simulink model "Energy_Management"  (R2025a)
settings: Solver=ode23tb  StartTime=0.0  StopTime=0.5  MaxStep=1e-5  RelTol=1e-3
undefined symbols (not defined in the file): Ion, Lithium
libraries: eeDiscretePi x7, spsSeriesRLCBranchLib x7, spsCurrentMeasurementLib x4, spsIGBTDiodeLib x4, spsPWMGeneratorDCDCLib x3, spsVoltageMeasurementLib x3, spsDiodeLib x2, spsBatteryLib x1, spsFuelCellStackLib x1, spsPVArrayLib x1, spsPWMGenerator2LevelLib x1, spsSeriesRLCLoadLib x1
settings Model: Creator=devin  LastModifiedBy=devin

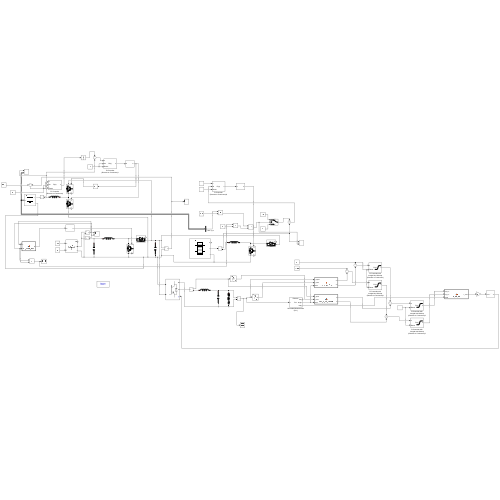
[thumbnail: Simulink's stored preview of the top-level diagram]
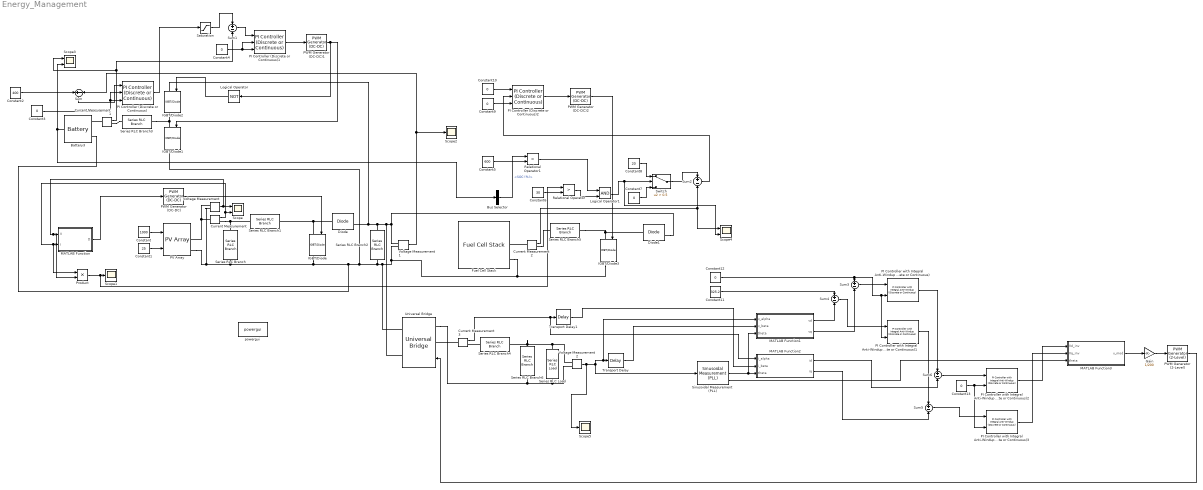
== system Energy_Management ==
  Battery3 : spsBatteryLib/Battery  BatType=Lithium-Ion  NomV=300  NomQ=48  SOC=100  Batt_Tr=45  PresetModel=on  MaxQ=48  MinV=225  FullV=349.1961  Dis_rate=20.8696  R=0.0625  Normal_OP=43.4087  expZone="[324.1158      2.358261]"
  Bus Selector : BusSelector  OutputSignals=SOC (%)
  Constant : Constant  Value=1000
  Constant1 : Constant  Value=25
  Constant{3..4,7,9..10,12..13} (7 alike) : Constant  Value=0
  Constant11 : Constant  Value=325.2
  Constant2 : Constant  Value=400
  Constant5 : Constant  Value=600
  Constant6 : Constant  Value=30
  Constant8 : Constant  Value=20
  Current Measurement{,1..3} (4 alike) : spsCurrentMeasurementLib/Current Measurement  PhasorSimulation=off  OutputType=Complex  PSBequivalent=0
  Diode : spsDiodeLib/Diode  Ron=0.001  Lon=0  Vf=0.8  IC=0  UseSnubber=0  Rs=500  Cs=250e-9  Measurements=on
  Diode1 : spsDiodeLib/Diode  Ron=0.001  Lon=0  Vf=0.8  IC=0  UseSnubber=0  Rs=500  Cs=250e-9  Measurements=on
  Fuel Cell Stack : spsFuelCellStackLib/Fuel Cell Stack  PresetModel=No (User-Defined)  FcType=0  Detailed=Detailed  Eoc=[330, 300]  NomVI=[20, 220]  EndVI=[35, 200]  Nc=315  n=55  TOp=65  AirFr=300  SuppPress=[1.5,1]  Comp=[99.95,21,1]  SignX=off  SignY=off  FlowRateH2=off  FlowRateAir=off  SystemTemp=off  SystemPH2=off  SystemPAir=off  FCDyn=off  FC_tau=1  Peak_O2=80  V_Under=10
      settings: LibrarySourceBlock=sps_lib/Sources/Fuel Cell Stack
  Gain : Gain  Gain=1/200
  IGBT/Diode{,1..3} (4 alike) : spsIGBTDiodeLib/IGBT//Diode  Ron=1e-3  Rs=1e5  Cs=inf  Measurements=on
  Logical Operator : Logic  Operator=NOT  AllPortsSameDT=off  OutDataTypeStr=boolean
  Logical Operator1 : Logic  AllPortsSameDT=off  OutDataTypeStr=boolean
  MATLAB Function : MATLAB Function  TreatAsAtomicUnit=on
  MATLAB Function1 : MATLAB Function  TreatAsAtomicUnit=on
  MATLAB Function2 : MATLAB Function  TreatAsAtomicUnit=on
  MATLAB Function3 : MATLAB Function  TreatAsAtomicUnit=on
  PI Controller (Discrete or Continuous) : eeDiscretePi/PI Controller (Discrete or Continuous)  Kp=0.1  Ki=5  Kaw=1  x0=0  Ts=-1
      settings: LibrarySourceBlock=|
      | ee_sl_lib/General Control/PI Controller
      | (Discrete or Continuous)
  PI Controller (Discrete or Continuous)1 : eeDiscretePi/PI Controller (Discrete or Continuous)  Kp=0.1  Ki=5  Kaw=1  x0=0  Ts=-1
      settings: LibrarySourceBlock=|
      | ee_sl_lib/General Control/PI Controller
      | (Discrete or Continuous)
  PI Controller (Discrete or Continuous)2 : eeDiscretePi/PI Controller (Discrete or Continuous)  Kp=0.2  Ki=20  Kaw=1  x0=0  Ts=-1
      settings: LibrarySourceBlock=|
      | ee_sl_lib/General Control/PI Controller
      | (Discrete or Continuous)
  PI Controller with Integral Anti-Windup (Discrete or Continuous) : eeDiscretePi/PI Controller with Integral Anti-Windup (Discrete or Continuous)  Kp=0.2  Ki=25  x0=0  B=15  A=-15  Ts=-1
      settings: LibrarySourceBlock=|
      | ee_sl_lib/General Control/PI Controller with
      | Integral Anti-Windup
      | (Discrete or Continuous)
  PI Controller with Integral Anti-Windup (Discrete or Continuous)1 : eeDiscretePi/PI Controller with Integral Anti-Windup (Discrete or Continuous)  Kp=0.2  Ki=25  x0=0  B=15  A=-15  Ts=-1
      settings: LibrarySourceBlock=|
      | ee_sl_lib/General Control/PI Controller with
      | Integral Anti-Windup
      | (Discrete or Continuous)
  PI Controller with Integral Anti-Windup (Discrete or Continuous)2 : eeDiscretePi/PI Controller with Integral Anti-Windup (Discrete or Continuous)  Kp=0.4  Ki=40  x0=0  B=0.95  A=-0.95  Ts=-1
      settings: LibrarySourceBlock=|
      | ee_sl_lib/General Control/PI Controller with
      | Integral Anti-Windup
      | (Discrete or Continuous)
  PI Controller with Integral Anti-Windup (Discrete or Continuous)3 : eeDiscretePi/PI Controller with Integral Anti-Windup (Discrete or Continuous)  Kp=0.4  Ki=40  x0=0  B=0.95  A=-0.95  Ts=-1
      settings: LibrarySourceBlock=|
      | ee_sl_lib/General Control/PI Controller with
      | Integral Anti-Windup
      | (Discrete or Continuous)
  PV Array : spsPVArrayLib/PV Array  Npar=1  Nser=8  PlotType=array @ 1000 W/m2 & specified temperatures  S_vec="[ 1000  500  100 ]"  Temp_C_vec="[ 45 25  ]"  ModuleName=User-defined  PlotWhenSelected=off  Pm=250.205  Ncell=60  Voc=37.8  Isc=8.75  Vm=30.7  Im=8.15  beta_Voc_pc=-0.36099  alpha_Isc_pc=0.102  beta_Voc=-0.13645  alpha_Isc=0.008925  IL=8.764  I0=3.2541e-10  nI=1.0219  Rsh=197.3099  Rs=0.29997  RobustModel=off  RobustCellTemperature=313.3991  BAL=on  Tc=1e-6  Tfilter=5e-5
  PWM Generator (2-Level) : spsPWMGenerator2LevelLib/PWM Generator (2-Level)  ModulatorType=Single-phase full-bridge - Bipolar modulation (4 pulses)  ModulatorMode=Unsynchronized  Fc=1000  Pc=90  nF=27  MinMax="[ -1  1 ]"  SamplingTechnique=Natural  ModulatingSignals=off  m=0.8  Freq=60  Phase=0  Ts=0  ShowCarrierOutport=off
  PWM Generator (DC-DC) : spsPWMGeneratorDCDCLib/PWM Generator (DC-DC)  Fsw=20000  Ts=0
  PWM Generator (DC-DC)1 : spsPWMGeneratorDCDCLib/PWM Generator (DC-DC)  Fsw=20000  Ts=0
  PWM Generator (DC-DC)2 : spsPWMGeneratorDCDCLib/PWM Generator (DC-DC)  Fsw=20000  Ts=0
  Product : Product
  Relational Operator : RelationalOperator  Operator=>  OutDataTypeStr=boolean  RndMeth=Simplest  InputSameDT=off
  Relational Operator1 : RelationalOperator  Operator=>  OutDataTypeStr=boolean  RndMeth=Simplest  InputSameDT=off
  Saturation : Saturate  UpperLimit=0.95  LowerLimit=0.05
  Scope : Scope  NumInputPorts=2
      settings: ActiveDisplayYMinimum=-32.437505931636437  ActiveDisplayYMaximum=299.72938020086377
  Scope1 : Scope
      settings: ActiveDisplayYMinimum=-250.09653918436439  ActiveDisplayYMaximum=2251.6858311968886
  Scope2 : Scope
      settings: ActiveDisplayYMinimum=327.296191460694  ActiveDisplayYMaximum=408.0782422570619  DataLoggingVariableName=ScopeData2
  Scope3 : Scope  NumInputPorts=2
      settings: ActiveDisplayYMinimum=-49.354169180280678  ActiveDisplayYMaximum=395.26293627147709  DataLoggingVariableName=ScopeData3
  Scope4 : Scope  NumInputPorts=2
      settings: ActiveDisplayYMinimum=-0.17740712010289458  ActiveDisplayYMaximum=0.30140270835281957  DataLoggingVariableName=ScopeData4
  Scope5 : Scope
      settings: ActiveDisplayYMinimum=-2463.1886461096151  ActiveDisplayYMaximum=2405.0943637829546  DataLoggingVariableName=ScopeData5
  Series RLC Branch : spsSeriesRLCBranchLib/Series RLC Branch  LConnTagsString=__new0  RConnTagsString=__new0  BranchType=C  Resistance=1  Inductance=1e-3  SetiL0=off  InitialCurrent=0  Capacitance=470e-6  Setx0=off  InitialVoltage=0  Measurements=None
  Series RLC Branch1 : spsSeriesRLCBranchLib/Series RLC Branch  LConnTagsString=__new0  RConnTagsString=__new0  BranchType=L  Resistance=1  Inductance=1e-3  SetiL0=off  InitialCurrent=0  Capacitance=1e-6  Setx0=off  InitialVoltage=0  Measurements=None
  Series RLC Branch2 : spsSeriesRLCBranchLib/Series RLC Branch  LConnTagsString=__new0  RConnTagsString=__new0  BranchType=C  Resistance=1  Inductance=1e-3  SetiL0=off  InitialCurrent=0  Capacitance=2200e-6  Setx0=on  InitialVoltage=400  Measurements=None
  Series RLC Branch3 : spsSeriesRLCBranchLib/Series RLC Branch  LConnTagsString=__new0  RConnTagsString=__new0  BranchType=L  Resistance=1  Inductance=2e-3  SetiL0=off  InitialCurrent=0  Capacitance=1e-6  Setx0=off  InitialVoltage=0  Measurements=None
  Series RLC Branch4 : spsSeriesRLCBranchLib/Series RLC Branch  LConnTagsString=__new0  RConnTagsString=__new0  BranchType=L  Resistance=1  Inductance=2e-3  SetiL0=off  InitialCurrent=0  Capacitance=1e-6  Setx0=off  InitialVoltage=0  Measurements=None
  Series RLC Branch5 : spsSeriesRLCBranchLib/Series RLC Branch  LConnTagsString=__new0  RConnTagsString=__new0  BranchType=L  Resistance=1  Inductance=1e-3  SetiL0=off  InitialCurrent=0  Capacitance=1e-6  Setx0=off  InitialVoltage=0  Measurements=None
  Series RLC Branch6 : spsSeriesRLCBranchLib/Series RLC Branch  LConnTagsString=__new0  RConnTagsString=__new0  BranchType=C  Resistance=1  Inductance=2e-3  SetiL0=off  InitialCurrent=0  Capacitance=10e-6  Setx0=off  InitialVoltage=0  Measurements=None
  Series RLC Load : spsSeriesRLCLoadLib/Series RLC Load  LConnTagsString=a  RConnTagsString=__new0  NominalVoltage=230  NominalFrequency=50  ActivePower=1200  InductivePower=100  CapacitivePower=100  Setx0=off  InitialVoltage=0  SetiL0=off  InitialCurrent=0  Measurements=None  LoadType=constant Z
  Sinusoidal Measurement (PLL) : eeSinusoidalMeasurementV2/Sinusoidal Measurement (PLL)  Ki_PD=1000  Kp_LF=400  Ki_LF=20000  F0=50  Theta0=0  Mag0=1  Ts=1e-6
      settings: LibrarySourceBlock=|
      | ee_sl_lib/Measurements/Sinusoidal Measurement
      | (PLL)
  Sum{,1..6} (7 alike) : Sum  Inputs=+-
  Switch : Switch  Criteria=u2 > Threshold  Threshold=0.5  SaturateOnIntegerOverflow=off  InputSameDT=off
  Transport Delay : TransportDelay  DelayTime=0.005  BufferSize=8192
  Transport Delay1 : TransportDelay  DelayTime=0.005  BufferSize=8192
  Universal Bridge : spsUniversalBridgeLib/Universal Bridge  Arms=2  SnubberResistance=1e5  SnubberCapacitance=inf  Device=IGBT / Diodes  Ron=1e-3  Lon=0  ForwardVoltages="[  0  0  ]"  ForwardVoltage=0  GTOparameters=[ 10e-6 , 20e-6 ]  IGBTparameters=[ 1e-6 , 2e-6 ]  Measurements=None  Measurements_2=None  converterType=Rectifier
  Voltage Measurement : spsVoltageMeasurementLib/Voltage Measurement  PhasorSimulation=off  OutputType=Complex  PSBequivalent=0
  Voltage Measurement1 : spsVoltageMeasurementLib/Voltage Measurement  PhasorSimulation=off  OutputType=Complex  PSBequivalent=0
  Voltage Measurement2 : spsVoltageMeasurementLib/Voltage Measurement  PhasorSimulation=off  OutputType=Complex  PSBequivalent=0
  powergui : sps_lib/powergui  Priority=1  SimulationMode=Discrete  SampleTime=1e-6  frequency=60  Iterations=50  frequencyindice=0  Pbase=100e6  ErrMax=1e-4  UnitsV=kV  UnitsW=MW  buscounter=0  FunctionMessages=off  echomessages=off  EnableUseOfTLC=off  CurrentSourceSwitches=off  DisableSnubberDevices=off  DisableRonSwitches=off  DisableVfSwitches=off  DisplayEquations=off  AutomaticDiscreteSolvers=off  SolverType=Tustin/Backward Euler (TBE)  Interpol=off  ExternalGateDelay=off  methode=off  Ts=100  x0status=blocks  SPID=on  SwTol=0  HookPort=off  NonlinearTolerance=1e-4  nMaxIteration=100  ContinueOnMaxIteration=off  RestoreLinks=warning  ResistiveCurrentMeasurement=off  Frange=[0:2:500]  Ylog=off  Xlog=on  ShowGrid=off  save=off  variable=ZData  structure=0  ZoomFFT=off  StartTime=0.0  cycles=1  DisplayStyle=1  fundamental=60  FreqAxis=off  MaxFrequency=1000  frequencyindicesteady=1  RmsSteady=1  display=off
  wires:
  Voltage Measurement/1 -> Product/2, MATLAB Function/1(V), Scope/1
  Current Measurement/1 -> Product/1, MATLAB Function/2(I), Scope/2
  MATLAB Function/1(D) -> PWM Generator (DC-DC)/1
  PWM Generator (DC-DC)/1 -> IGBT/Diode/1
  Constant/1 -> PV Array/1
  Constant1/1 -> PV Array/2
  Constant2/1 -> Sum/1
  Voltage Measurement1/1 -> Sum/2, Scope2/1
  Sum/1 -> PI Controller (Discrete or Continuous)/1
  PI Controller (Discrete or Continuous)/1 -> Saturation/1
  PWM Generator (DC-DC)1/1 -> Logical Operator/1, IGBT/Diode1/1
  Logical Operator/1 -> IGBT/Diode2/1
  Constant3/1 -> PI Controller (Discrete or Continuous)/3, PI Controller (Discrete or Continuous)/2
  Saturation/1 -> Sum1/1
  Current Measurement1/1 -> Sum1/2, Scope3/1
  PI Controller (Discrete or Continuous)1/1 -> PWM Generator (DC-DC)1/1
  Sum1/1 -> PI Controller (Discrete or Continuous)1/1
  Constant4/1 -> PI Controller (Discrete or Continuous)1/2, PI Controller (Discrete or Continuous)1/3
  Product/1 -> Relational Operator/1, Scope1/1
  Bus Selector/1 -> Relational Operator1/1  "<SOC (%)>"
  Relational Operator1/1 -> Logical Operator1/1
  Relational Operator/1 -> Logical Operator1/2
  Logical Operator1/1 -> Switch/2, Scope4/2
  Constant8/1 -> Switch/1
  Constant7/1 -> Switch/3
  Switch/1 -> Sum2/1
  Current Measurement2/1 -> Scope4/1, Sum2/2
  Sum2/1 -> PI Controller (Discrete or Continuous)2/2
  PI Controller (Discrete or Continuous)2/1 -> PWM Generator (DC-DC)2/1
  PWM Generator (DC-DC)2/1 -> IGBT/Diode3/1
  Constant6/1 -> Relational Operator/2
  Constant5/1 -> Relational Operator1/2
  Constant10/1 -> PI Controller (Discrete or Continuous)2/1
  Constant9/1 -> PI Controller (Discrete or Continuous)2/3
  Voltage Measurement2/1 -> Scope5/1, Sinusoidal Measurement (PLL)/1, MATLAB Function1/1(v_alpha), Transport Delay/1
  Transport Delay/1 -> MATLAB Function1/2(v_beta)
  Current Measurement3/1 -> MATLAB Function2/1(i_alpha), Transport Delay1/1
  MATLAB Function1/1(vd) -> Sum4/2
  Constant11/1 -> Sum4/1
  Constant12/1 -> PI Controller with Integral Anti-Windup (Discrete or Continuous)1/2, PI Controller with Integral Anti-Windup (Discrete or Continuous)/2, Sum3/1
  MATLAB Function1/2(vq) -> Sum3/2
  Sum3/1 -> PI Controller with Integral Anti-Windup (Discrete or Continuous)/1
  Sum4/1 -> PI Controller with Integral Anti-Windup (Discrete or Continuous)1/1
  Transport Delay1/1 -> MATLAB Function2/2(i_beta)
  Sinusoidal Measurement (PLL)/2 -> MATLAB Function2/3(theta), MATLAB Function1/3(theta)
  PI Controller with Integral Anti-Windup (Discrete or Continuous)/1 -> Sum6/1
  PI Controller with Integral Anti-Windup (Discrete or Continuous)1/1 -> Sum5/1
  MATLAB Function2/1(id) -> Sum6/2
  MATLAB Function2/2(iq) -> Sum5/2
  Sum6/1 -> PI Controller with Integral Anti-Windup (Discrete or Continuous)2/1
  Sum5/1 -> PI Controller with Integral Anti-Windup (Discrete or Continuous)3/1
  PI Controller with Integral Anti-Windup (Discrete or Continuous)2/1 -> MATLAB Function3/1(Vd_inv)
  PI Controller with Integral Anti-Windup (Discrete or Continuous)3/1 -> MATLAB Function3/2(Vq_inv)
  Sinusoidal Measurement (PLL)/3 -> MATLAB Function3/3(theta)
  MATLAB Function3/1(v_mod) -> Gain/1
  Gain/1 -> PWM Generator (2-Level)/1
  Constant13/1 -> PI Controller with Integral Anti-Windup (Discrete or Continuous)2/2, PI Controller with Integral Anti-Windup (Discrete or Continuous)3/2
  PWM Generator (2-Level)/1 -> Universal Bridge/1
  Battery3/1 -> Scope3/2, Bus Selector/1
  connections:
  Series RLC Branch1/LConn1 -- Current Measurement/RConn1 -- Series RLC Branch/LConn1
  PV Array/RConn2 -- Battery3/LConn2 -- Series RLC Branch2/RConn1 -- Universal Bridge/RConn2 -- Fuel Cell Stack/RConn2 -- IGBT/Diode3/RConn1 -- Voltage Measurement1/LConn2 -- IGBT/Diode1/RConn1 -- IGBT/Diode/RConn1 -- Series RLC Branch/RConn1 -- Voltage Measurement/LConn2
  IGBT/Diode/LConn1 -- Diode/LConn1 -- Series RLC Branch1/RConn1
  Diode/RConn1 -- IGBT/Diode2/LConn1 -- Universal Bridge/RConn1 -- Diode1/RConn1 -- Voltage Measurement1/LConn1 -- Series RLC Branch2/LConn1
  Current Measurement/LConn1 -- Voltage Measurement/LConn1 -- PV Array/RConn1
  IGBT/Diode1/LConn1 -- Series RLC Branch3/LConn1 -- IGBT/Diode2/RConn1
  Current Measurement1/LConn1 -- Battery3/LConn1
  Current Measurement1/RConn1 -- Series RLC Branch3/RConn1
  Series RLC Branch5/RConn1 -- Diode1/LConn1 -- IGBT/Diode3/LConn1
  Current Measurement2/LConn1 -- Fuel Cell Stack/RConn1
  Current Measurement2/RConn1 -- Series RLC Branch5/LConn1
  Current Measurement3/LConn1 -- Universal Bridge/LConn1
  Series RLC Branch4/LConn1 -- Current Measurement3/RConn1
  Series RLC Branch6/LConn1 -- Voltage Measurement2/LConn1 -- Series RLC Load/LConn1 -- Series RLC Branch4/RConn1
  Universal Bridge/LConn2 -- Series RLC Load/RConn1 -- Voltage Measurement2/LConn2 -- Series RLC Branch6/RConn1

== matlab function Energy_Management/MATLAB Function1 ==
  data: v_alpha input; vd output; v_beta input; theta input; vq output
function [vd, vq] = abc_to_dq_voltage(v_alpha, v_beta, theta)
    vd =  v_alpha * cos(theta) + v_beta * sin(theta);
    vq = -v_alpha * sin(theta) + v_beta * cos(theta);
end

== matlab function Energy_Management/MATLAB Function ==
  data: V input; D output; I input
function D = inc_cond_mppt(V, I)
    % Persistent variables retain their state across simulation time steps
    persistent Vold Iold Dold;
    
    % Initialize variables on the very first time step
    if isempty(Vold)
        Vold = V;
        Iold = I;
        Dold = 0.45; % Starting duty cycle near midpoint
    end
    
    % Step size parameter - determines tracking speed and steady-state ripple
    deltaD = 0.0005; 
    
    % Calculate instantaneous changes
    dV = V - Vold;
    dI = I - Iold;
    
    % Incremental Conductance core tracking logic
    if dV == 0
        if dI > 0
            Dold = Dold - deltaD; % Increase voltage by dropping duty cycle
        elseif dI < 0
            Dold = Dold + deltaD; % Decrease voltage by increasing duty cycle
        end
    else
        % Check if the incremental conductance equals instantaneous conductance
        if (dI / dV) == (-I / V)
            % System is exactly at MPP; maintain current duty cycle
        elseif (dI / dV) > (-I / V)
            Dold = Dold - deltaD; % Left of MPP: Decrease D to ramp up V_pv
        else
            Dold = Dold + deltaD; % Right of MPP: Increase D to drop V_pv
        end
    end
    
    % Hardware constraints: Limit duty cycle safely between 10% and 85%
    if Dold > 0.85
        Dold = 0.85;
    elseif Dold < 0.10
        Dold = 0.10;
    end
    
    % Pass duty cycle to output port and save values for next iteration
    D = Dold;
    Vold = V;
    Iold = I;
end

== matlab function Energy_Management/MATLAB Function2 ==
  data: i_alpha input; id output; i_beta input; theta input; iq output
function [id, iq] = abc_to_dq_current(i_alpha, i_beta, theta)
    id =  i_alpha * cos(theta) + i_beta * sin(theta);
    iq = -i_alpha * sin(theta) + i_beta * cos(theta);
end

== matlab function Energy_Management/MATLAB Function3 ==
  data: Vd_inv input; v_mod output; Vq_inv input; theta input
function v_mod = dq_to_abc(Vd_inv, Vq_inv, theta)
    % Convert back to alpha-beta reference frame
    v_alpha_star = Vd_inv * cos(theta) - Vq_inv * sin(theta);

    % In a single-phase system, the alpha component is your actual modulating wave
    v_mod = v_alpha_star;
end
